simulink model "LoopShapingLead"  (R2017a)
settings: Solver=ode45  StartTime=0.0  StopTime=5  RelTol=1e-3  EnableMultiTasking=on
values from neighbouring files (symbols this model uses):
  G_LoSim = G_LoVar(k)    [LoopShaping_TP.m]
  m = 0.5    [LCS_freq.m]    (also in LoopShaping_TP.m = 2)
  w_pSim = w_pVar(1,k)    [LoopShaping_TP.m]
  w_zSim = w_zVar(1,k)    [LoopShaping_TP.m]
settings Model: Creator=Kathleeen  LastModifiedBy=kathleen
settings DataIOCC: LimitDataPoints=on  SaveFormat=Array
settings OptimizationCC: LifeSpan=inf
settings DebuggingCC: UnderspecifiedInitializationDetection=Classic  MergeDetectMultiDrivingBlocksExec=none  StateNameClashWarn=warning  SFUnexpectedBacktrackingDiag=warning  SFNoUnconditionalDefaultTransitionDiag=warning  SFExecutionAtInitializationDiag=none
settings HardwareCC: ProdBitPerPointer=32  ProdBitPerSizeT=32  ProdBitPerPtrDiffT=32  ProdLargestAtomicFloat=None  ProdIntDivRoundTo=Undefined  ProdEndianess=Unspecified  ProdWordSize=32  ProdHWDeviceType=32-bit Generic
settings ModelReferenceCC: PropagateSignalLabelsOutOfModel=off
settings GRTTargetCC: TargetLangStandard=C89/C90 (ANSI)  GeneratePreprocessorConditionals=Disable all
settings ConfigComp: CovMetricSettings=dw  CovHtmlReporting=on  CovSaveCumulativeToWorkspaceVar=on  CovSaveSingleToWorkspaceVar=on  CovExternalEMLEnable=off

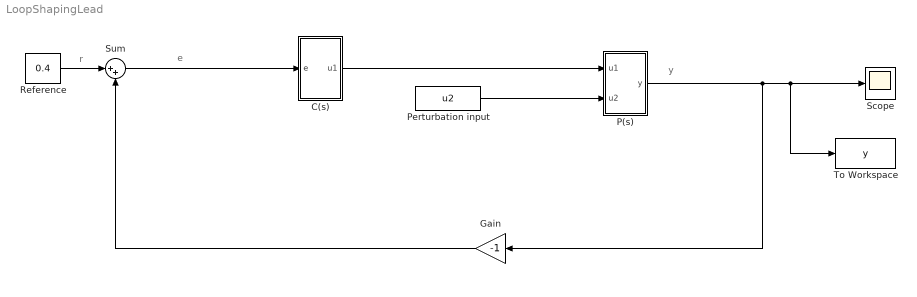
== system LoopShapingLead ==
  note: e
  note: r
  note: y
  C(s) : Subsystem
  Gain : Gain  Gain=-1
  P(s) : Subsystem
  Perturbation input : FromWorkspace  VariableName=u2  SampleTime=0
  Reference : Constant  Value=0.4
  Scope : Scope
  Sum : Sum  Inputs=|++
  To Workspace : ToWorkspace  VariableName=y  SaveFormat=Timeseries  SampleTime=-1
  wires:
  Gain/1 -> Sum/2
  Reference/1 -> Sum/1
  Sum/1 -> C(s)/1(e)
  C(s)/1(u1) -> P(s)/1(u1)
  Perturbation input/1 -> P(s)/2(u2)
  P(s)/1(y) -> Gain/1, To Workspace/1, Scope/1

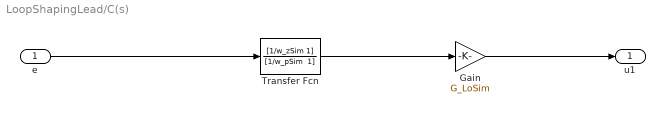
== system LoopShapingLead/C(s) ==
  e : Inport
  Gain : Gain  Gain=G_LoSim
  Transfer Fcn : TransferFcn  Numerator=[1/w_zSim 1]  Denominator="[1/w_pSim  1]"
  u1 : Outport
  wires:
  Gain/1 -> u1/1
  e/1 -> Transfer Fcn/1
  Transfer Fcn/1 -> Gain/1

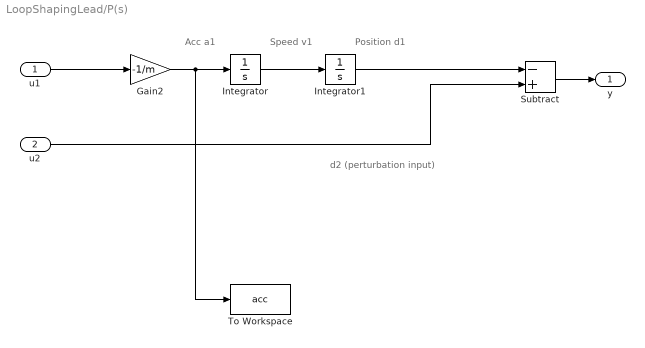
== system LoopShapingLead/P(s) ==
  note: d2 (perturbation input)
  note: Position d1
  note: Speed v1
  note: Acc a1
  u1 : Inport
  u2 : Inport  Port=2
  Gain2 : Gain  Gain=-1/m
  Integrator : Integrator
  Integrator1 : Integrator
  Subtract : Sum  Inputs=-+
  To Workspace : ToWorkspace  VariableName=acc  SaveFormat=Timeseries  SampleTime=-1
  y : Outport
  wires:
  u1/1 -> Gain2/1
  Subtract/1 -> y/1
  u2/1 -> Subtract/2
  Gain2/1 -> To Workspace/1, Integrator/1
  Integrator/1 -> Integrator1/1
  Integrator1/1 -> Subtract/1
